simulink model "modele_pure_gain_regulator"  (Simulink 7.1)
settings: Solver=ode45  StartTime=0.0  StopTime=2  RelTol=1e-3
undefined symbols (not defined in the file or in its folder): Ac, Kc
settings Model: Creator=ahp  LastModifiedBy=ahp

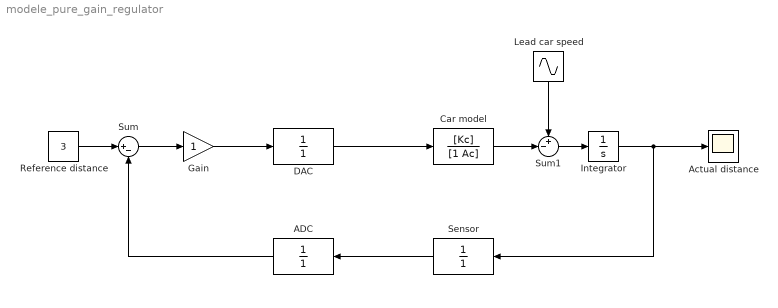
== system modele_pure_gain_regulator ==
  ADC : TransferFcn  Orientation=left  Denominator=[1]
  Actual distance : Scope
  Car model : TransferFcn  Numerator=[Kc]  Denominator=[1 Ac]
  DAC : TransferFcn  Denominator=[1]
  Gain : Gain  ParameterDataType=sfix(16)  ParameterScaling=2^0  OutDataType=sfix(16)  OutScaling=2^0
  Integrator : Integrator
  Lead car speed : Sin  Orientation=down  SampleTime=0
  Reference distance : Constant  Value=3  OutDataType=sfix(16)  OutScaling=2^0
  Sensor : TransferFcn  Orientation=left  Denominator=[1]
  Sum : Sum  Inputs=|+-  OutDataType=sfix(16)  OutScaling=2^0
  Sum1 : Sum  Inputs=+-|  OutDataType=sfix(16)  OutScaling=2^0
  wires:
  Reference distance/1 -> Sum/1
  Sum/1 -> Gain/1
  Car model/1 -> Sum1/2
  Lead car speed/1 -> Sum1/1
  Sum1/1 -> Integrator/1
  Integrator/1 -> Actual distance/1, Sensor/1
  ADC/1 -> Sum/2
  Gain/1 -> DAC/1
  DAC/1 -> Car model/1
  Sensor/1 -> ADC/1
